simulink model "ROSCO"  (R2019a)
settings: Solver=ode4  StartTime=0.0  StopTime=TMax  FixedStep=dt  RelTol=1e-3  EnableMultiTasking=on
values from neighbouring files (symbols this model uses):
  ContParam = Pre_ContParam_TSR_NREL5MW    [run_ROSCO.m]
  cpscan = Pre_LoadRotPerf(txtfile)    [run_ROSCO.m]
  dt = FastIn.DT    [run_ROSCO.m]
  FastIn = Pre_SimSetup(ModDir, ModName, ElastoFile)    [run_ROSCO.m]
  OutList = Post_LoadOutlist(SFunc_OutfileName)    [run_ROSCO.m]
  TSR_opt = TSRvec(Cpvec == max(Cpvec))    [run_ROSCO.m]
undefined symbols (not defined in the file or in its folder): DiscIntNeverNeededParam, Filt, strmatch
libraries: simulink x6
settings Model: Creator=nabbas  LastModifiedBy=nabbas
settings DataIOCC: SaveTime=off  ReturnWorkspaceOutputs=off
settings DebuggingCC: ArithmeticOperatorsInVariantConditions=warning
settings SFSimCC: SimUseLocalCustomCode=off
settings RTWCC: RTWUseLocalCustomCode=off
settings CodeAppCC: StateflowObjectComments=on

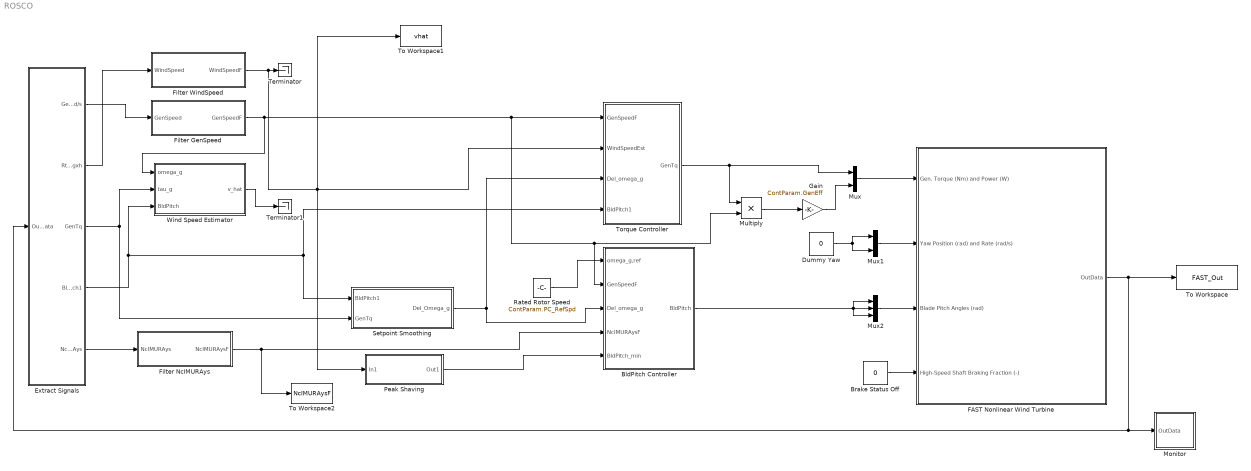
== system ROSCO ==
  BldPitch Controller : Subsystem
  Brake Status Off : Constant  Value=0
  Dummy Yaw : Constant  Value=0
  Extract Signals : Subsystem  TreatAsAtomicUnit=on
  FAST Nonlinear Wind Turbine : Subsystem  mask(FAST Nonlinear Wind Turbine){}
      mask help: This block contains the FAST S-Function.
      mask init:
      | clear FAST_SFunc
  Filter GenSpeed : Subsystem
  Filter NcIMURAys : Subsystem
  Filter WindSpeed : Subsystem
  Gain : Gain  Gain=ContParam.GenEff
  Monitor : Subsystem  TreatAsAtomicUnit=on
  Multiply : Product
  Mux : Mux  Inputs=2
  Mux1 : Mux  Inputs=2
  Mux2 : Mux  Inputs=3
  Peak Shaving : Subsystem
  Rated Rotor Speed : Constant  Value=ContParam.PC_RefSpd
  Setpoint Smoothing : Subsystem
  Terminator : Terminator
  Terminator1 : Terminator
  To Workspace : ToWorkspace  VariableName=FAST_Out  SaveFormat=Timeseries  SampleTime=-1
  To Workspace1 : ToWorkspace  VariableName=vhat  SaveFormat=Timeseries  SampleTime=-1
  To Workspace2 : ToWorkspace  VariableName=NcIMURAysF  SaveFormat=Timeseries  SampleTime=-1
  Torque Controller : Subsystem
  Wind Speed Estimator : Subsystem
  wires:
  FAST Nonlinear Wind Turbine/1(OutData) -> Monitor/1(OutData), Extract Signals/1(OutData), To Workspace/1
  Dummy Yaw/1 -> Mux1/2, Mux1/1
  Mux1/1 -> FAST Nonlinear Wind Turbine/2(Yaw Position (rad) and Rate (rad/s))
  Mux2/1 -> FAST Nonlinear Wind Turbine/3(Blade Pitch Angles (rad))
  BldPitch Controller/1(BldPitch) -> Mux2/3, Mux2/1, Mux2/2
  Brake Status Off/1 -> FAST Nonlinear Wind Turbine/4(High-Speed Shaft Braking Fraction (-))
  Filter GenSpeed/1(GenSpeedF) -> Wind Speed Estimator/1(omega_g), Torque Controller/1(GenSpeedF), Multiply/2, BldPitch Controller/2(GenSpeedF)
  Mux/1 -> FAST Nonlinear Wind Turbine/1(Gen. Torque (Nm) and Power (W))
  Extract Signals/1(GenSpeed_rad/s) -> Filter GenSpeed/1(GenSpeed)
  Extract Signals/4(BldPitch1) -> Wind Speed Estimator/3(BldPitch), Torque Controller/4(BldPitch1), Setpoint Smoothing/1(BldPitch1)
  Extract Signals/3(GenTq) -> Wind Speed Estimator/2(tau_g), Setpoint Smoothing/2(GenTq)
  Setpoint Smoothing/1(Del_Omega_g) -> BldPitch Controller/3(Del_omega_g), Torque Controller/3(Del_omega_g)
  Rated Rotor Speed/1 -> BldPitch Controller/1(omega_g,ref)
  Gain/1 -> Mux/2
  Extract Signals/2(RtVAvgxh) -> Filter WindSpeed/1(WindSpeed)
  Extract Signals/5(NcIMURAys) -> Filter NcIMURAys/1(NcIMURAys)
  Filter NcIMURAys/1(NcIMURAysF) -> To Workspace2/1, BldPitch Controller/4(NcIMURAysF)
  Peak Shaving/1(Out1) -> BldPitch Controller/5(BldPitch_min)
  Torque Controller/1(GenTq) -> Mux/1, Multiply/1
  Multiply/1 -> Gain/1
  Filter WindSpeed/1(WindSpeedF) -> To Workspace1/1, Torque Controller/2(WindSpeedEst), Peak Shaving/1(In1), Terminator/1
  Wind Speed Estimator/1(v_hat) -> Terminator1/1

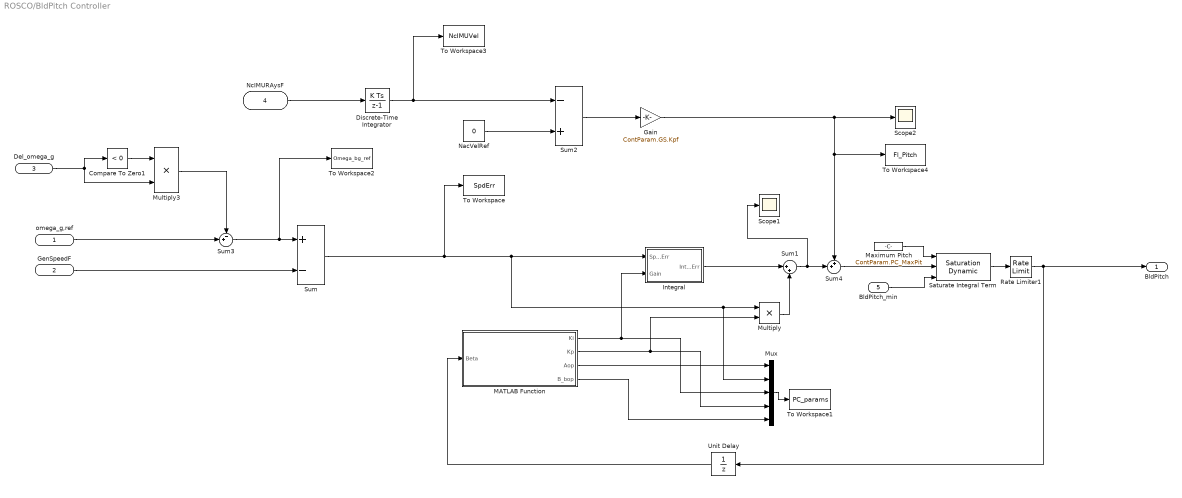
== system ROSCO/BldPitch Controller ==
  omega_g,ref : Inport
  GenSpeedF : Inport  Port=2
  Del_omega_g : Inport  Port=3
  NcIMURAysF : Inport  Port=4
  BldPitch_min : Inport  Port=5
  Compare To Zero1 : simulink/Logic and Bit Operations/Compare To Zero  relop=<  OutDataTypeStr=boolean
  Discrete-Time Integrator : DiscreteIntegrator  gainval=1  SampleTime=-1  ICPrevOutput=DiscIntNeverNeededParam  ICPrevScaledInput=DiscIntNeverNeededParam
  Gain : Gain  Gain=ContParam.GS.Kpf
  Integral : Subsystem
  MATLAB Function : MATLAB Function  TreatAsAtomicUnit=on
  Maximum Pitch : Constant  Value=ContParam.PC_MaxPit
  Multiply : Product
  Multiply3 : Product
  Mux : Mux  Inputs=5
  NacVelRef : Constant  Value=0
  Rate Limiter1 : RateLimiter  RisingSlewLimit=ContParam.PC_MaxRat  FallingSlewLimit=-ContParam.PC_MaxRat  SampleTimeMode=inherited  InitialCondition=FastIn.BlPitch1*pi/180
  Saturate Integral Term : simulink/Discontinuities/Saturation Dynamic  OutMin=[]  OutMax=ContParam.PC_MaxPit  OutDataTypeStr=Inherit: Same as second input  OutDataType=fixdt(1, 16)  OutScaling=2^-10  RndMeth=Nearest  DoSatur=off
  Scope1 : Scope
  Scope2 : Scope
  Sum : Sum  Inputs=+-
  Sum1 : Sum  Inputs=|++
  Sum2 : Sum  Inputs=-+
  Sum3 : Sum  Inputs=-+|
  Sum4 : Sum  Inputs=++|
  To Workspace : ToWorkspace  VariableName=SpdErr  SaveFormat=Timeseries  SampleTime=-1
  To Workspace1 : ToWorkspace  VariableName=PC_params  SaveFormat=Structure  SampleTime=-1
  To Workspace2 : ToWorkspace  VariableName=Omega_bg_ref  SaveFormat=Timeseries  SampleTime=-1
  To Workspace3 : ToWorkspace  VariableName=NcIMUVel  SaveFormat=Timeseries  SampleTime=-1
  To Workspace4 : ToWorkspace  VariableName=Fl_Pitch  SaveFormat=Timeseries  SampleTime=-1
  Unit Delay : UnitDelay  InitialCondition=FastIn.BlPitch1 * pi/180  SampleTime=-1  HasFrameUpgradeWarning=on
  BldPitch : Outport
  wires:
  Multiply/1 -> Sum1/2
  Integral/1(IntSpdErr) -> Sum1/1
  MATLAB Function/1(Ki) -> Mux/3, Integral/2(Gain)
  MATLAB Function/2(Kp) -> Mux/4, Multiply/2
  Mux/1 -> To Workspace1/1
  Saturate Integral Term/1 -> Rate Limiter1/1
  MATLAB Function/3(Aop) -> Mux/1
  Sum/1 -> To Workspace/1, Mux/2, Multiply/1, Integral/1(SpeedErr)
  Rate Limiter1/1 -> Unit Delay/1, BldPitch/1
  Sum3/1 -> To Workspace2/1, Sum/1
  GenSpeedF/1 -> Sum/2
  Compare To Zero1/1 -> Multiply3/1
  Del_omega_g/1 -> Compare To Zero1/1, Multiply3/2
  Multiply3/1 -> Sum3/1
  Unit Delay/1 -> MATLAB Function/1(Beta)
  Sum1/1 -> Scope1/1, Sum4/2
  MATLAB Function/4(B_bop) -> Mux/5
  omega_g,ref/1 -> Sum3/2
  Sum4/1 -> Saturate Integral Term/2
  BldPitch_min/1 -> Saturate Integral Term/3
  Maximum Pitch/1 -> Saturate Integral Term/1
  NacVelRef/1 -> Sum2/2
  Sum2/1 -> Gain/1
  NcIMURAysF/1 -> Discrete-Time Integrator/1
  Gain/1 -> To Workspace4/1, Sum4/1, Scope2/1
  Discrete-Time Integrator/1 -> Sum2/1, To Workspace3/1

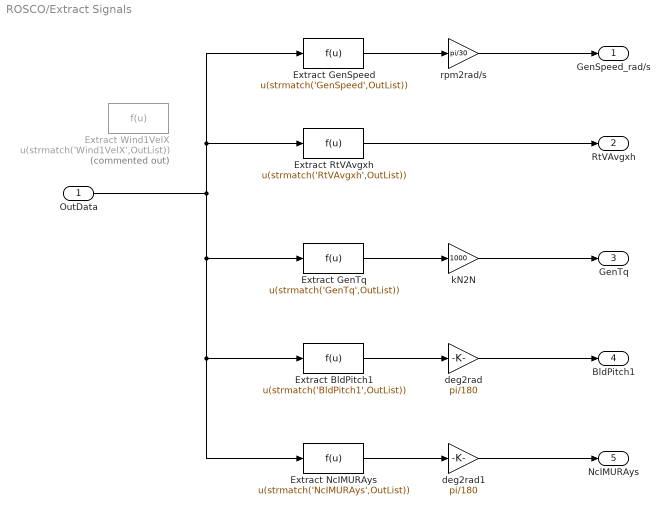
== system ROSCO/Extract Signals ==
  OutData : Inport
  Extract BldPitch1 : Fcn  Expr=u(strmatch('BldPitch1',OutList))
  Extract GenSpeed : Fcn  Expr=u(strmatch('GenSpeed',OutList))
  Extract GenTq : Fcn  Expr=u(strmatch('GenTq',OutList))
  Extract NcIMURAys : Fcn  Expr=u(strmatch('NcIMURAys',OutList))
  Extract RtVAvgxh : Fcn  Expr=u(strmatch('RtVAvgxh',OutList))
  Extract Wind1VelX : Fcn  Commented=on  Expr=u(strmatch('Wind1VelX',OutList))
  deg2rad : Gain  Gain=pi/180
  deg2rad1 : Gain  Gain=pi/180
  kN2N : Gain  Gain=1000
  rpm2rad/s : Gain  Gain=pi/30
  GenSpeed_rad/s : Outport
  RtVAvgxh : Outport  Port=2
  GenTq : Outport  Port=3
  BldPitch1 : Outport  Port=4
  NcIMURAys : Outport  Port=5
  wires:
  Extract RtVAvgxh/1 -> RtVAvgxh/1
  Extract GenSpeed/1 -> rpm2rad/s/1
  rpm2rad/s/1 -> GenSpeed_rad/s/1
  Extract BldPitch1/1 -> deg2rad/1
  deg2rad/1 -> BldPitch1/1
  Extract GenTq/1 -> kN2N/1
  kN2N/1 -> GenTq/1
  deg2rad1/1 -> NcIMURAys/1
  Extract NcIMURAys/1 -> deg2rad1/1
  OutData/1 -> Extract RtVAvgxh/1, Extract GenSpeed/1, Extract NcIMURAys/1, Extract BldPitch1/1, Extract GenTq/1

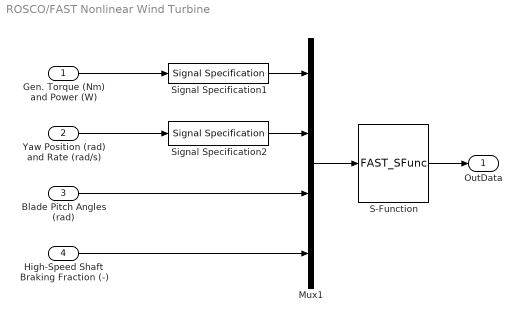
== system ROSCO/FAST Nonlinear Wind Turbine ==
  Gen. Torque (Nm) and Power (W) : Inport
  Yaw Position (rad) and Rate (rad/s) : Inport  Port=2
  Blade Pitch Angles (rad) : Inport  Port=3
  High-Speed Shaft Braking Fraction (-) : Inport  Port=4
  Mux1 : Mux
  S-Function : S-Function  FunctionName=FAST_SFunc  Parameters=FAST_InputFileName, TMax, 0  SFunctionDeploymentMode=off  EnableBusSupport=off
  Signal Specification1 : SignalSpecification  OutDataTypeStr=double  Dimensions=2
  Signal Specification2 : SignalSpecification  OutDataTypeStr=double  Dimensions=2
  OutData : Outport
  wires:
  Gen. Torque (Nm) and Power (W)/1 -> Signal Specification1/1
  S-Function/1 -> OutData/1
  Mux1/1 -> S-Function/1
  Blade Pitch Angles (rad)/1 -> Mux1/3
  Yaw Position (rad) and Rate (rad/s)/1 -> Signal Specification2/1
  Signal Specification1/1 -> Mux1/1
  Signal Specification2/1 -> Mux1/2
  High-Speed Shaft Braking Fraction (-)/1 -> Mux1/4

== system ROSCO/Filter GenSpeed ==
  GenSpeed : Inport
  Discrete Filter : DiscreteFilter  Numerator=Filt.HSS.b  Denominator=Filt.HSS.a  InitialStates=ContParam.PC_Vrated
  First-Order LPF : Subsystem
  Second-Order LPF : Subsystem  Commented=on
  To Workspace2 : ToWorkspace  VariableName=Om_f  SaveFormat=Timeseries  SampleTime=-1
  GenSpeedF : Outport
  wires:
  GenSpeed/1 -> Discrete Filter/1
  Discrete Filter/1 -> To Workspace2/1, GenSpeedF/1

== system ROSCO/Filter NcIMURAys ==
  NcIMURAys : Inport
  Discrete Filter : DiscreteFilter  Numerator=Filt.Floating.b  Denominator=Filt.Floating.a  InitialStatesSource=Input port
      settings: InputPortMap=u0,p5
  Discrete Filter1 : DiscreteFilter  Numerator=Filt.Fl2.b  Denominator=Filt.Fl2.a  InitialStatesSource=Input port
      settings: InputPortMap=u0,p5
  NcIMURAysF : Outport
  wires:
  NcIMURAys/1 -> Discrete Filter/1, Discrete Filter/2
  Discrete Filter/1 -> Discrete Filter1/1, Discrete Filter1/2
  Discrete Filter1/1 -> NcIMURAysF/1

== system ROSCO/Filter WindSpeed ==
  WindSpeed : Inport
  Discrete Filter : DiscreteFilter  Numerator=Filt.Wind.b  Denominator=Filt.Wind.a  InitialStates=ContParam.PC_Vrated
  To Workspace2 : ToWorkspace  VariableName=WindSpeedF  SaveFormat=Timeseries  SampleTime=-1
  WindSpeedF : Outport
  wires:
  Discrete Filter/1 -> WindSpeedF/1, To Workspace2/1
  WindSpeed/1 -> Discrete Filter/1

== system ROSCO/Monitor ==
  OutData : Inport
  Extract BldPitch1 : Fcn  Expr=u(strmatch('BldPitch1',OutList))
  Extract GenTq : Fcn  Expr=u(strmatch('GenTq',OutList))
  Extract RotSpeed : Fcn  Expr=u(strmatch('RotSpeed',OutList))
  Scope : Scope  NumInputPorts=3
  wires:
  Extract BldPitch1/1 -> Scope/3
  OutData/1 -> Extract RotSpeed/1, Extract BldPitch1/1, Extract GenTq/1
  Extract RotSpeed/1 -> Scope/1
  Extract GenTq/1 -> Scope/2

== system ROSCO/Peak Shaving ==
  In1 : Inport
  Discrete Filter : DiscreteFilter  Numerator=Filt.PeakShaving.b  Denominator=Filt.PeakShaving.a
  PeakShaving : MATLAB Function  TreatAsAtomicUnit=on
  Out1 : Outport
  wires:
  In1/1 -> Discrete Filter/1
  Discrete Filter/1 -> PeakShaving/1(v_est)
  PeakShaving/1(Beta_min) -> Out1/1

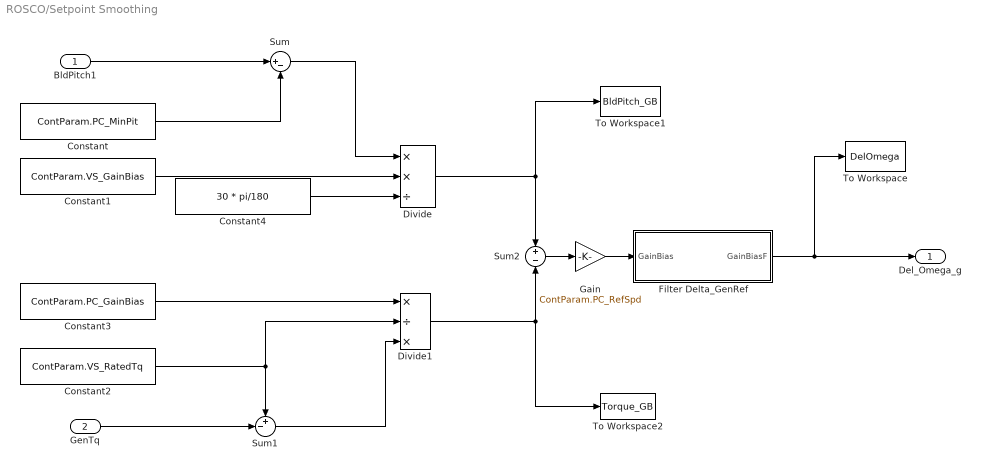
== system ROSCO/Setpoint Smoothing ==
  BldPitch1 : Inport
  GenTq : Inport  Port=2
  Constant : Constant  Value=ContParam.PC_MinPit
  Constant1 : Constant  Value=ContParam.VS_GainBias
  Constant2 : Constant  Value=ContParam.VS_RatedTq
  Constant3 : Constant  Value=ContParam.PC_GainBias
  Constant4 : Constant  Value=30 * pi/180
  Divide : Product  Inputs=**/
  Divide1 : Product  Inputs=*/*
  Filter Delta_GenRef : Subsystem
  Gain : Gain  Gain=ContParam.PC_RefSpd
  Sum : Sum  Inputs=|+-
  Sum1 : Sum  Inputs=+-|
  Sum2 : Sum  Inputs=+|-
  To Workspace : ToWorkspace  VariableName=DelOmega  SaveFormat=Timeseries  SampleTime=-1
  To Workspace1 : ToWorkspace  VariableName=BldPitch_GB  SaveFormat=Timeseries  SampleTime=-1
  To Workspace2 : ToWorkspace  VariableName=Torque_GB  SaveFormat=Timeseries  SampleTime=-1
  Del_Omega_g : Outport
  wires:
  GenTq/1 -> Sum1/2
  Constant2/1 -> Sum1/1, Divide1/2
  Constant/1 -> Sum/2
  Sum1/1 -> Divide1/3
  Sum2/1 -> Gain/1
  BldPitch1/1 -> Sum/1
  Sum/1 -> Divide/1
  Constant1/1 -> Divide/2
  Constant3/1 -> Divide1/1
  Constant4/1 -> Divide/3
  Filter Delta_GenRef/1(GainBiasF) -> Del_Omega_g/1, To Workspace/1
  Divide/1 -> To Workspace1/1, Sum2/1
  Divide1/1 -> To Workspace2/1, Sum2/2
  Gain/1 -> Filter Delta_GenRef/1(GainBias)

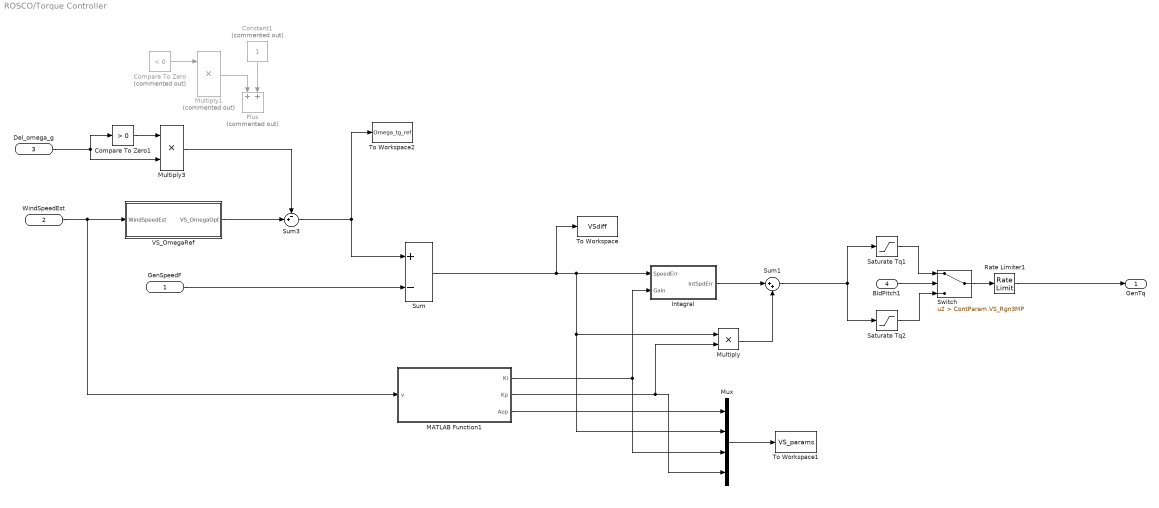
== system ROSCO/Torque Controller ==
  GenSpeedF : Inport
  WindSpeedEst : Inport  Port=2
  Del_omega_g : Inport  Port=3
  BldPitch1 : Inport  Port=4
  Compare To Zero : simulink/Logic and Bit Operations/Compare To Zero  Commented=on  relop=<  OutDataTypeStr=boolean
  Compare To Zero1 : simulink/Logic and Bit Operations/Compare To Zero  relop=>  OutDataTypeStr=boolean
  Constant1 : Constant  Commented=on
  Integral : Subsystem
  MATLAB Function1 : MATLAB Function  TreatAsAtomicUnit=on
  Multiply : Product
  Multiply1 : Product  Commented=on
  Multiply3 : Product
  Mux : Mux
  Plus : Sum  Commented=on
  Rate Limiter1 : RateLimiter  RisingSlewLimit=ContParam.VS_MaxRat  FallingSlewLimit=-ContParam.VS_MaxRat  SampleTimeMode=inherited
  Saturate Tq1 : Saturate  UpperLimit=ContParam.VS_RatedTq  LowerLimit=-ContParam.VS_MaxTq
  Saturate Tq2 : Saturate  UpperLimit=ContParam.VS_RatedTq  LowerLimit=-ContParam.VS_MaxTq
  Sum : Sum  Inputs=+-
  Sum1 : Sum  Inputs=|++
  Sum3 : Sum  Inputs=-+|
  Switch : Switch  Criteria=u2 > Threshold  Threshold=ContParam.VS_Rgn3MP
  To Workspace : ToWorkspace  VariableName=VSdiff  SaveFormat=Timeseries  SampleTime=-1
  To Workspace1 : ToWorkspace  VariableName=VS_params  SaveFormat=Structure  SampleTime=-1
  To Workspace2 : ToWorkspace  VariableName=Omega_tg_ref  SaveFormat=Timeseries  SampleTime=-1
  VS_OmegaRef : Subsystem
  GenTq : Outport
  wires:
  Multiply/1 -> Sum1/2
  Integral/1(IntSpdErr) -> Sum1/1
  MATLAB Function1/1(Ki) -> Mux/3, Integral/2(Gain)
  MATLAB Function1/2(Kp) -> Multiply/2, Mux/4
  Mux/1 -> To Workspace1/1
  VS_OmegaRef/1(VS_OmegaOpt) -> Sum3/2
  GenSpeedF/1 -> Sum/2
  MATLAB Function1/3(Aop) -> Mux/1
  WindSpeedEst/1 -> MATLAB Function1/1(v), VS_OmegaRef/1(WindSpeedEst)
  Compare To Zero/1 -> Multiply1/1
  Sum3/1 -> To Workspace2/1, Sum/1
  Rate Limiter1/1 -> GenTq/1
  Sum/1 -> To Workspace/1, Integral/1(SpeedErr), Multiply/1, Mux/2
  Sum1/1 -> Saturate Tq2/1, Saturate Tq1/1
  Saturate Tq2/1 -> Switch/3
  Switch/1 -> Rate Limiter1/1
  Saturate Tq1/1 -> Switch/1
  BldPitch1/1 -> Switch/2
  Multiply1/1 -> Plus/1
  Constant1/1 -> Plus/2
  Compare To Zero1/1 -> Multiply3/1
  Del_omega_g/1 -> Compare To Zero1/1, Multiply3/2
  Multiply3/1 -> Sum3/1

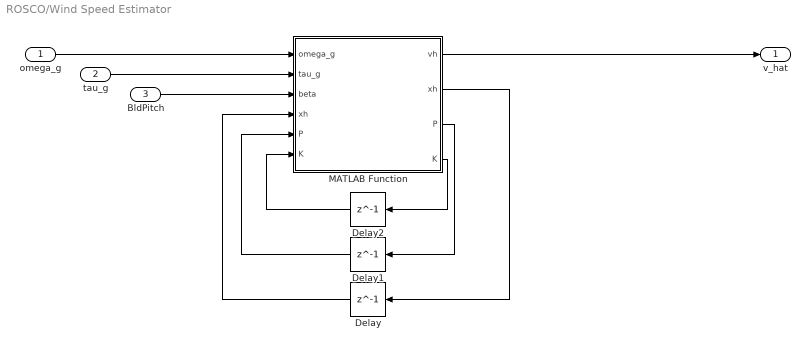
== system ROSCO/Wind Speed Estimator ==
  omega_g : Inport
  tau_g : Inport  Port=2
  BldPitch : Inport  Port=3
  Delay : Delay  DelayLength=1  InitialCondition=[FastIn.RotSpeed*pi/30, 0, ContParam.WSE_v0]'
  Delay1 : Delay  DelayLength=1  InitialCondition=diag([0.1, 0.1, 1])^2
  Delay2 : Delay  DelayLength=1  InitialCondition=zeros(3,1)
  MATLAB Function : MATLAB Function  TreatAsAtomicUnit=on
  v_hat : Outport
  wires:
  MATLAB Function/2(xh) -> Delay/1
  Delay/1 -> MATLAB Function/4("xh ")
  MATLAB Function/3(P) -> Delay1/1
  Delay1/1 -> MATLAB Function/5("P ")
  omega_g/1 -> MATLAB Function/1(omega_g)
  tau_g/1 -> MATLAB Function/2(tau_g)
  BldPitch/1 -> MATLAB Function/3(beta)
  MATLAB Function/4(K) -> Delay2/1
  Delay2/1 -> MATLAB Function/6("K ")
  MATLAB Function/1(vh) -> v_hat/1

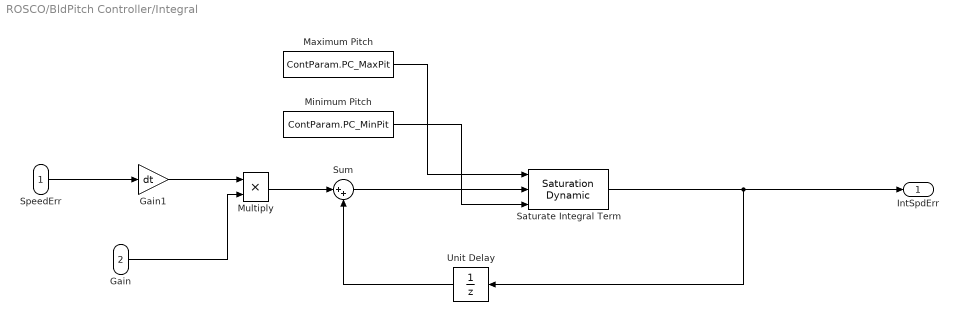
== system ROSCO/BldPitch Controller/Integral ==
  SpeedErr : Inport
  Gain : Inport  Port=2
  Gain1 : Gain  Gain=dt
  Maximum Pitch : Constant  Value=ContParam.PC_MaxPit
  Minimum Pitch : Constant  Value=ContParam.PC_MinPit
  Multiply : Product
  Saturate Integral Term : simulink/Discontinuities/Saturation Dynamic  OutMin=[]  OutMax=[]  OutDataTypeStr=Inherit: Same as second input  OutDataType=fixdt(1, 16)  OutScaling=2^-10  RndMeth=Nearest  DoSatur=off
  Sum : Sum  Inputs=|++
  Unit Delay : UnitDelay  InitialCondition=FastIn.BlPitch1 * pi/180  SampleTime=-1  HasFrameUpgradeWarning=on
  IntSpdErr : Outport
  wires:
  Maximum Pitch/1 -> Saturate Integral Term/1
  Unit Delay/1 -> Sum/2
  Minimum Pitch/1 -> Saturate Integral Term/3
  Sum/1 -> Saturate Integral Term/2
  SpeedErr/1 -> Gain1/1
  Gain/1 -> Multiply/2
  Saturate Integral Term/1 -> IntSpdErr/1, Unit Delay/1
  Gain1/1 -> Multiply/1
  Multiply/1 -> Sum/1

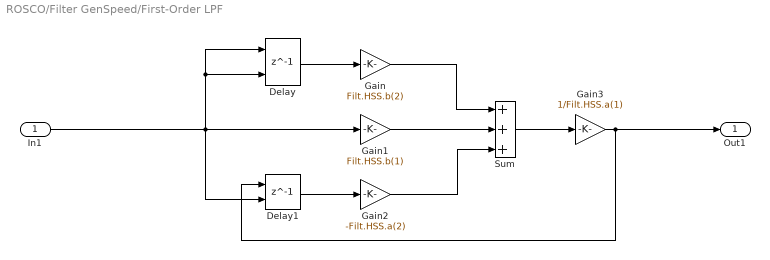
== system ROSCO/Filter GenSpeed/First-Order LPF ==
  In1 : Inport
  Delay : Delay  DelayLength=1  InitialConditionSource=Input port  InitialCondition=FastIn.RotSpeed * ContParam.GBRatio * pi/30
      settings: InputPortMap=u0,p4
  Delay1 : Delay  DelayLength=1  InitialConditionSource=Input port  InitialCondition=FastIn.RotSpeed * ContParam.GBRatio * pi/30
      settings: InputPortMap=u0,p4
  Gain : Gain  Gain=Filt.HSS.b(2)
  Gain1 : Gain  Gain=Filt.HSS.b(1)
  Gain2 : Gain  Gain=-Filt.HSS.a(2)
  Gain3 : Gain  Gain=1/Filt.HSS.a(1)
  Sum : Sum  Inputs=+++
  Out1 : Outport
  wires:
  Gain3/1 -> Out1/1, Delay1/1
  Gain2/1 -> Sum/3
  Gain/1 -> Sum/1
  Sum/1 -> Gain3/1
  Gain1/1 -> Sum/2
  In1/1 -> Delay1/2, Gain1/1, Delay/2, Delay/1
  Delay1/1 -> Gain2/1
  Delay/1 -> Gain/1

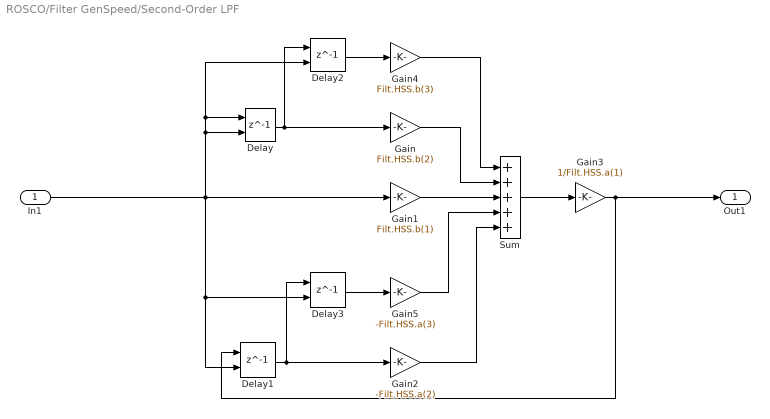
== system ROSCO/Filter GenSpeed/Second-Order LPF ==
  In1 : Inport
  Delay{,1..3} (4 alike) : Delay  DelayLength=1  InitialConditionSource=Input port  InitialCondition=FastIn.RotSpeed * ContParam.GBRatio * pi/30
      settings: InputPortMap=u0,p4
  Gain : Gain  Gain=Filt.HSS.b(2)
  Gain1 : Gain  Gain=Filt.HSS.b(1)
  Gain2 : Gain  Gain=-Filt.HSS.a(2)
  Gain3 : Gain  Gain=1/Filt.HSS.a(1)
  Gain4 : Gain  Gain=Filt.HSS.b(3)
  Gain5 : Gain  Gain=-Filt.HSS.a(3)
  Sum : Sum  Inputs=+++++
  Out1 : Outport
  wires:
  Delay/1 -> Delay2/1, Gain/1
  Delay1/1 -> Delay3/1, Gain2/1
  In1/1 -> Delay2/2, Delay/1, Delay/2, Gain1/1, Delay1/2, Delay3/2
  Gain1/1 -> Sum/3
  Sum/1 -> Gain3/1
  Gain/1 -> Sum/2
  Gain2/1 -> Sum/5
  Gain3/1 -> Delay1/1, Out1/1
  Delay3/1 -> Gain5/1
  Gain5/1 -> Sum/4
  Gain4/1 -> Sum/1
  Delay2/1 -> Gain4/1

== system ROSCO/Setpoint Smoothing/Filter Delta_GenRef ==
  GainBias : Inport
  Discrete Filter : DiscreteFilter  Numerator=Filt.GBFilt.b  Denominator=Filt.GBFilt.a
  GainBiasF : Outport
  wires:
  GainBias/1 -> Discrete Filter/1
  Discrete Filter/1 -> GainBiasF/1

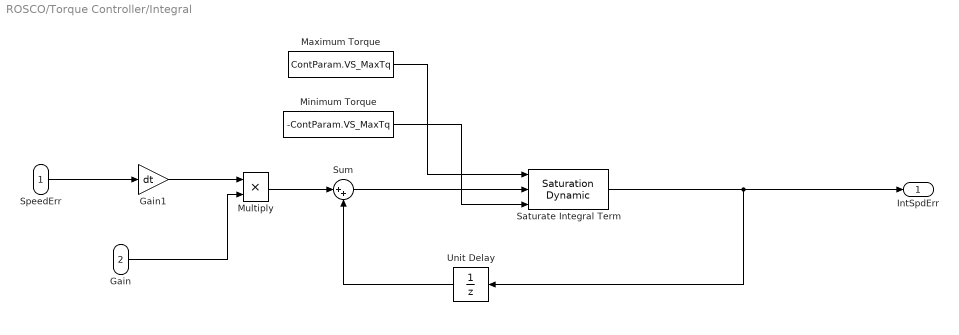
== system ROSCO/Torque Controller/Integral ==
  SpeedErr : Inport
  Gain : Inport  Port=2
  Gain1 : Gain  Gain=dt
  Maximum Torque : Constant  Value=ContParam.VS_MaxTq
  Minimum Torque : Constant  Value=-ContParam.VS_MaxTq
  Multiply : Product
  Saturate Integral Term : simulink/Discontinuities/Saturation Dynamic  OutMin=[]  OutMax=[]  OutDataTypeStr=Inherit: Same as second input  OutDataType=fixdt(1, 16)  OutScaling=2^-10  RndMeth=Nearest  DoSatur=off
  Sum : Sum  Inputs=|++
  Unit Delay : UnitDelay  InitialCondition=ContParam.VS_RatedTq  SampleTime=-1  HasFrameUpgradeWarning=on
  IntSpdErr : Outport
  wires:
  Maximum Torque/1 -> Saturate Integral Term/1
  Unit Delay/1 -> Sum/2
  Minimum Torque/1 -> Saturate Integral Term/3
  Sum/1 -> Saturate Integral Term/2
  SpeedErr/1 -> Gain1/1
  Gain/1 -> Multiply/2
  Saturate Integral Term/1 -> IntSpdErr/1, Unit Delay/1
  Gain1/1 -> Multiply/1
  Multiply/1 -> Sum/1

== system ROSCO/Torque Controller/VS_OmegaRef ==
  WindSpeedEst : Inport
  Omega_opt : Subsystem
  Reference TSR : Constant  Value=TSR_opt
  Saturation : Saturate  UpperLimit=ContParam.PC_RefSpd  LowerLimit=FastIn.RotSpeed * 30/pi
  To Workspace1 : ToWorkspace  VariableName=Om_opt  SaveFormat=Timeseries  SampleTime=-1
  VS_OmegaOpt : Outport
  wires:
  WindSpeedEst/1 -> Omega_opt/2(Wind Speed)
  Omega_opt/1(Omega_opt) -> Saturation/1
  Reference TSR/1 -> Omega_opt/1(TSR_opt)
  Saturation/1 -> VS_OmegaOpt/1, To Workspace1/1

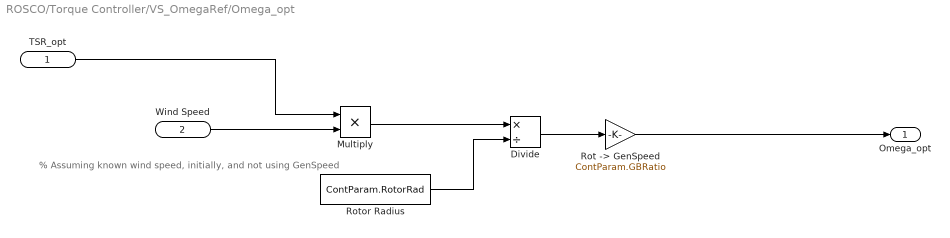
== system ROSCO/Torque Controller/VS_OmegaRef/Omega_opt ==
  note: % Assuming known wind speed, initially, and not using GenSpeed
  TSR_opt : Inport
  Wind Speed : Inport  Port=2
  Divide : Product  Inputs=*/
  Multiply : Product
  "Rot -> GenSpeed" : Gain  Gain=ContParam.GBRatio
  Rotor Radius : Constant  Value=ContParam.RotorRad
  Omega_opt : Outport
  wires:
  TSR_opt/1 -> Multiply/1
  Wind Speed/1 -> Multiply/2
  Multiply/1 -> Divide/1
  Rotor Radius/1 -> Divide/2
  Divide/1 -> "Rot -> GenSpeed"/1
  "Rot -> GenSpeed"/1 -> Omega_opt/1

== matlab function ROSCO/Wind Speed Estimator/MATLAB Function ==
  data: omega_g input; tau_g input; beta input; vh output; xh input; P input; K input; xh output; P output; ContParam parameter; FastIn parameter; cpscan parameter; K output
function [vh,xh,P,K] = WSE_EKF(omega_g, tau_g, beta, xh, P, K, ContParam, FastIn, cpscan)
% This function defines a WSE based off of an Extended Kalman Filter
% Inputs:
% Outputs:
% Nikhar Abbas

% Load ContParam variables
J = ContParam.J;                    % Rotor Inertia
rho = ContParam.rho;                % Air density
Rr = ContParam.RotorRad;             % Rotor Radius, R
A = pi*Rr^2;                         % Rotor Swept Area, m^2
Ng = ContParam.GBRatio;             % Gearbox Ratio
dt = FastIn.DT;                     % Timestep size (s)
pA = ContParam.GS.pA;               % System pole fit
% Constants
H = [1 0 0];
R = 0.02;
L = 4 * ContParam.RotorRad;
tui = 0.2;
V22 = 2^2/600;

% F = [om_m(1), 0, v_n(1)];

% organize Inputs
om_r = xh(1);
v_t = xh(2);
v_m = xh(3);
om_m = omega_g  / Ng;

% Load Cp data
TSRvec = cpscan.TSR;
Betavec = cpscan.BlPitch .* pi/180;
Cpmat = cpscan.Cpmat;

% Find current estimated operating conditions, and saturate
v_r = v_t + v_m;
% v_r = max( min(v_r, vv(end)), vv(1));
TSRe = om_m*Rr/v_r; 
% TSRe = max( min(TSRe, TSRvec(end)), TSRvec(1));

% Find current Cp 
% CpTSR = zeros(1,length(TSRvec));
% for TSRi = 1:length(TSRvec)
%     CpTSR(TSRi) = interp1(Betavec, Cpmat(TSRi,:), beta); % Vector of Cp values corresponding to operational beta
% end
% Cp = interp1(TSRvec, CpTSR, TSRe) ;
Cp = interp2(Betavec, TSRvec, Cpmat, beta, TSRe);
Cp = max(0,Cp);

% Calculate Jacobians
Aop = interp1(ContParam.GS.vv, ContParam.GS.A, v_r);
F = [Aop, 1/(2*J)*rho*A*Cp*3*(v_m+v_t)^2*1/om_r, 1/(2*J)*rho*A*Cp*3*(v_m+v_t)^2*1/om_r;...   
    0, pi*v_m/(2*L), pi*v_t/(2*L);...
    0, 0, 0];

% F = [pA(1).*(v_m+v_t) + pA(2), 1/(2*J)*rho*A*Cp*3*(v_m+v_t)^2*1/om_r, 1/(2*J)*rho*A*Cp*3*(v_m+v_t)^2*1/om_r;...   
%     0, pi*v_m/(2*L), pi*v_t/(2*L);...
%     0, 0, 0];

% Update Covariance 
V11 = (pi * v_m^3 * tui^2) / L;
V = [V11 0; 0 V22];
Q = diag([1e-5, V11, V22]);


%% Prediction Update

% state
tau_r = 1/2*rho*A*Cp*v_r^3 * 1/(om_m);       % Torque calculation
a = pi*v_m/(2*L);                           % Wind variance
dom_r = 1/J * (tau_r - Ng*tau_g);
dv_t = -a*v_t;
dv_m = 0;
dxh = [dom_r; dv_t; dv_m];

xh = xh + dt*dxh;
% P = F*P*F' + Q; % EKF
dP = F*P + P*F' + Q - K*R*K';
P = P + dt*dP;

% y_til = om_m - om_r;
y_til = om_m - om_r;

%% Measurement Update
S = H*P*H' + R;
K = P*H'/S;

xh = xh + K*y_til;
P = (eye(3) - K*H)*P; %EKF
% P = P - K*S*K';
% P = (eye(3) - K*H)*P*(eye(3) - K*H)' + K*R*K'; 



% Find Wind Speed Estimate
vh = v_m + v_t;


end

== matlab function ROSCO/Peak Shaving/PeakShaving ==
  data: v_est input; Beta_min output; ContParam parameter
function Beta_min = PeakShaving(v_est,ContParam)

% Define minimum pitch angle for blade pitch controller
%
% Inputs: v_est  - estimated wind speed
%         ContParam - structure of controller parameters. Contains peak
%                     shaving schedule

% Load minimum pitch angle schedule
vv = ContParam.GS.vv;
Beta_min_lookup = ContParam.GS.Beta_min;

% Define minimum blade pitch
Beta_min = interp1(vv,Beta_min_lookup,v_est);

Beta_min = max(Beta_min, ContParam.PC_MinPit);

== matlab function ROSCO/BldPitch Controller/MATLAB Function ==
  data: Ki output; Beta input; Kp output; ContParam parameter; Aop output; B_bop output
% function [Ki, Kp, Aop, B_bop] = GainSchedule(v, ContParam)
function [Ki, Kp, Aop, B_bop] = GainSchedule(Beta, ContParam)

% This function calculates the current gains for a Collective Blade Pitch 
% controller
%
% Inputs: v - Current wind speed estimate, m/s.
%         ContParam - Structure of control parameters, output from
%                     ControlParameters.m
%
% Outputs: Kp - Proportional Gain
%          Ki - Integral Gain
%
% Nikhar Abbas - May 2019


%% Linear Gain Schedule
% pKp_pc = ContParam.GS.pKp_pc;
% pKi_pc = ContParam.GS.pKi_pc;
% 
% %%
% Kp = pKp_pc(1)*Beta + pKp_pc(2);
% Ki = pKi_pc(1)*Beta + pKi_pc(2);
% % Kp = pKp_pc(1)*v + pKp_pc(2)
% % Ki = pKi_pc(1)*v + pKi_pc(2);
% 
% Kpmax = pKp_pc(1)*15*pi/180 + pKp_pc(2);
% Kimax = pKi_pc(1)*15*pi/180 + pKi_pc(2);
% 
% Kp = min(Kp, Kpmax);
% Ki = min(Ki,Kimax);

%% nonlinear Gain Schedule
Kp_pc = ContParam.GS.Kp_pc;
Ki_pc = ContParam.GS.Ki_pc;
PC_beta = ContParam.GS.PC_beta;
beta = max(min(Beta,PC_beta(end)), PC_beta(1));

% gains
Kp = interp1(PC_beta,Kp_pc, beta);
Ki = interp1(PC_beta,Ki_pc, beta);

%% Remove this
Aop=0;
B_bop=0;


end

== matlab function ROSCO/Torque Controller/MATLAB Function1 ==
  data: Ki output; v input; ContParam parameter; Kp output; Aop output
function [Ki, Kp, Aop] = GainSchedule(v,ContParam)
% This function calculates the gains for a variable speed torque controller
% for the DTU 10MW Wind Turbine
%
% Inputs: v - estimated wind speed (m/s)
%         omega - Generator Speed (rad/s)
%         ContParam = Control parameters - from ControlParameters_TSR.m
%         Avec - Vector of system poles - from Pre_TSRtracking_Plant.m

% Outputs: Kp - Proportional Gain
%          Ki - Integral Gain
%          Aop - Saturated system pole
%
% Nikhar Abbas - May 2019

%% Linear Gain Schedule
% pKp_vs = ContParam.GS.pKp_vs;
% pKi_vs = ContParam.GS.pKi_vs;
% 
% Kp = pKp_vs(1)*v + pKp_vs(2);
% Ki = pKi_vs;
% 
% 
% Aop=0;

%% NonLinear Gain Schedule
Kp_vs = ContParam.GS.Kp_vs;
Ki_vs = ContParam.GS.Ki_vs;
vs_v = ContParam.GS.VS_vv;
v = max(min(v,vs_v(end)), vs_v(1));

% gains
Kp = interp1(vs_v,Kp_vs, v);
Ki = interp1(vs_v,Ki_vs, v);

Aop=0;


end
